simulink model "B_dot"  (R2022b)
settings: Solver=VariableStepAuto  StartTime=0.0  StopTime=12000  RelTol=1e-3
undefined symbols (not defined in the file or in its folder): magnetorquers, r0, sat, sensors, settings, v0
libraries: matrix_library x5, simulink x2, cstblocks x1
settings Model: Creator=robertopistonenascone  LastModifiedBy=robertopistonenascone

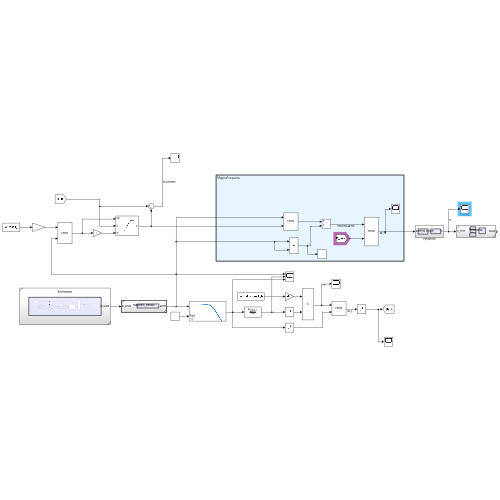
[thumbnail: Simulink's stored preview of the top-level diagram]
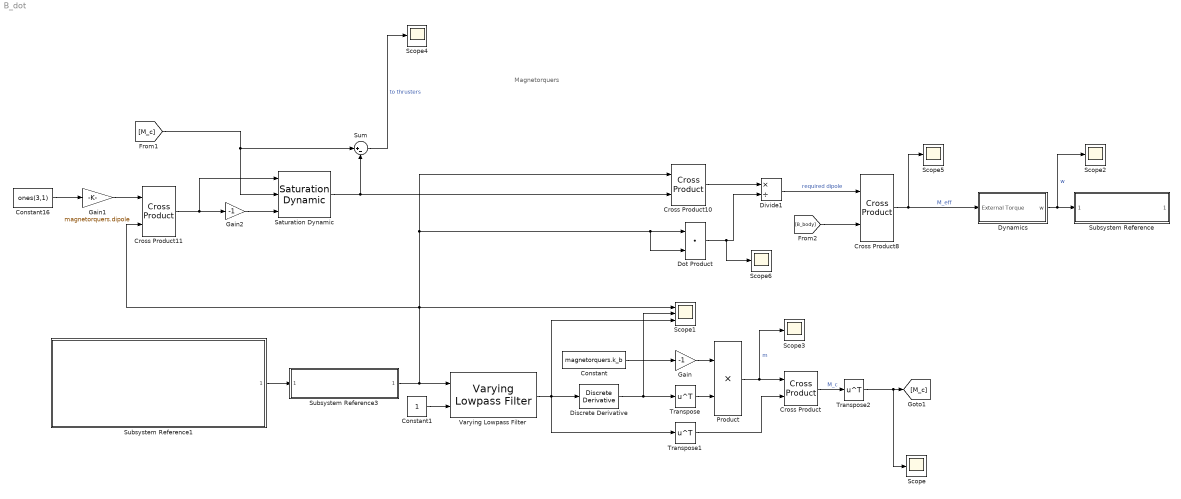
== system B_dot ==
  note: Magnetorquers
  Constant : Constant  Value=magnetorquers.k_b
  Constant1 : Constant
  Constant16 : Constant  Value=ones(3,1)
  Cross Product{,8,10..11} (4 alike) : matrix_library/Cross Product
  Discrete Derivative : simulink/Discrete/Discrete Derivative  gainval=1.0  ICPrevScaledInput=1e-4*[1 1 1]'  OutMin=[]  OutMax=[]  OutDataType=fixdt(1, 16)  OutScaling=2^-10  DoSatur=off
  Divide1 : Product  Inputs=*/  RndMeth=Zero  SaturateOnIntegerOverflow=on
  Dot Product : DotProduct  OutDataTypeStr=Inherit: Inherit via internal rule
  Dynamics : Subsystem
  Gain : Gain  Gain=-1
  Gain1 : Gain  Gain=magnetorquers.dipole
  Gain2 : Gain  Gain=-1
  Product : Product
  Saturation Dynamic : simulink/Discontinuities/Saturation Dynamic  OutMin=[]  OutMax=[]  OutDataTypeStr=Inherit: Same as second input  OutDataType=fixdt(1, 16)  OutScaling=2^-10  DoSatur=off
  Scope{,2..6} (6 alike) : Scope
  Scope1 : Scope  NumInputPorts=3
  Subsystem Reference : Subsystem  ReferencedSubsystem=Kinematics
  Subsystem Reference1 : Subsystem  ReferencedSubsystem=Enviroment
  Subsystem Reference3 : Subsystem  TreatAsAtomicUnit=on  SystemSampleTime=sensors.mag.frequency  ReferencedSubsystem=magnetic_sensor
  Sum : Sum  Inputs=|+-
  Transpose : Math  Operator=transpose
  Transpose1 : Math  Operator=transpose
  Transpose2 : Math  Operator=transpose
  Varying Lowpass Filter : cstblocks/Linear Parameter Varying/Varying Lowpass Filter  N=1
  wires:
  Gain/1 -> Product/1
  Constant/1 -> Gain/1
  Product/1 -> Cross Product/1, Scope3/1  "m"
  Discrete Derivative/1 -> Scope1/2, Transpose/1
  Transpose/1 -> Product/2
  Cross Product/1 -> Transpose2/1  "M_c"
  Subsystem Reference1/1 -> Subsystem Reference3/1
  Dynamics/1(w) -> Scope2/1, Subsystem Reference/1  "w"
  Constant1/1 -> Varying Lowpass Filter/2
  Transpose1/1 -> Cross Product/2
  Transpose2/1 -> Scope/1, [M_c]
  Subsystem Reference3/1 -> Cross Product11/2, Cross Product10/1, Dot Product/2, Dot Product/1, Scope1/1, Varying Lowpass Filter/1
  Cross Product11/1 -> Saturation Dynamic/1, Gain2/1
  Divide1/1 -> Cross Product8/1  "required dipole"
  Constant16/1 -> Gain1/1
  Cross Product10/1 -> Divide1/1
  [M_c] -> Saturation Dynamic/2, Sum/1
  Saturation Dynamic/1 -> Sum/2, Cross Product10/2
  Sum/1 -> Scope4/1  "to thrusters"
  Gain1/1 -> Cross Product11/1
  Varying Lowpass Filter/1 -> Transpose1/1, Discrete Derivative/1, Scope1/3
  Gain2/1 -> Saturation Dynamic/3
  [B_body] -> Cross Product8/2
  Cross Product8/1 -> Dynamics/1(External Torque), Scope5/1  "M_eff"
  Dot Product/1 -> Scope6/1, Divide1/2

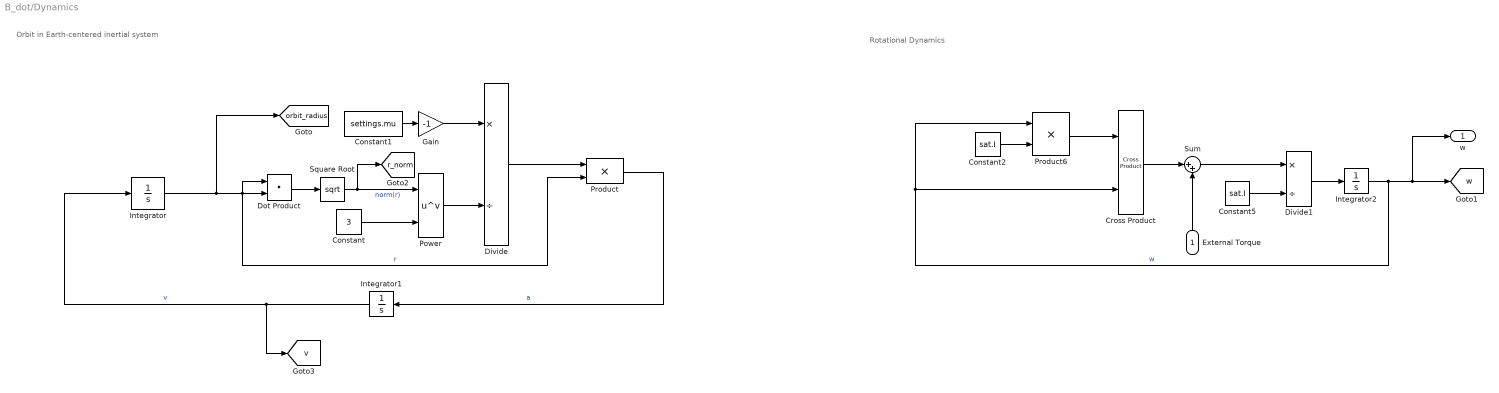
== system B_dot/Dynamics ==
  note: Rotational Dynamics
  note: Orbit in Earth-centered inertial system
  External Torque : Inport
  Constant : Constant  Value=3
  Constant1 : Constant  Value=settings.mu
  Constant2 : Constant  Value=sat.I
  Constant5 : Constant  Value=sat.I
  Cross Product : matrix_library/Cross Product
  Divide : Product  Inputs=*/
  Divide1 : Product  Inputs=*/
  Dot Product : DotProduct  OutDataTypeStr=Inherit: Inherit via internal rule
  Gain : Gain  Gain=-1
  Integrator : Integrator  InitialCondition=r0
  Integrator1 : Integrator  InitialCondition=v0
  Integrator2 : Integrator  InitialCondition=settings.w0
  Power : Math  Operator=pow
  Product : Product
  Product6 : Product
  Square Root : Sqrt
  Sum : Sum  Inputs=|++
  w : Outport
  tag scope: orbit_radius=global, r_norm=global, v=global, w=global
  wires:
  Constant/1 -> Power/2
  Integrator1/1 -> Integrator/1, [v]  "v"
  Dot Product/1 -> Square Root/1
  Square Root/1 -> [r_norm], Power/1  "norm(r)"
  Power/1 -> Divide/2
  Divide/1 -> Product/1
  Gain/1 -> Divide/1
  Integrator/1 -> [orbit_radius], Product/2, Dot Product/2, Dot Product/1  "r"
  Product/1 -> Integrator1/1  "a"
  Constant1/1 -> Gain/1
  Divide1/1 -> Integrator2/1
  Sum/1 -> Divide1/1
  Product6/1 -> Cross Product/1
  Integrator2/1 -> Cross Product/2, Product6/1, w/1, [w]  "w"
  Constant2/1 -> Product6/2
  Cross Product/1 -> Sum/1
  Constant5/1 -> Divide1/2
  External Torque/1 -> Sum/2
